simulink model "templateVFreplay"  (R2019b)
settings: Solver=ode23tb  StartTime=0  StopTime=dataSim(l).Time(end)  FixedStep=Ts
model workspace (MAT data in the model file):
  AC8B_test_sdosession : sldodialogs.data.SessionData (value not decoded)
  tp34291882_bceb_4da8_b486_81ba615ab517 = [0 0.0333333 0.0666667 0.1 0.1333334 0.1666667 0.2 0.2333333 0.2666666 0.2999999 0.3333332 0.3666665 ... (13500 elements, 2700x5)]
  tp5fd81924_c6b2_4820_a4c1_c746ac51258e : object (value not decoded)
  tp61e2f470_2812_498a_af75_e87b8b944307 = [0 0.0333333 0.0666667 0.1 0.1333334 0.1666667 0.2 0.2333333 0.2666666 0.2999999 0.3333332 0.3666665 ... (13500 elements, 2700x5)]
  tpfa3056f0_c430_45b3_969f_b76cef1498ad : object (value not decoded)
undefined symbols (not defined in the file): dataSim, dyn, Fnom, g, gcbh, genTpd0, genTppd0, genTppq0, genTpq0, genXd, genXl, genXpd, genXppd, genXppq, genXpq, genXq, govDisable, ifd, init, j, l, MBase, p, sps_rtmsupport, sys, Tb1, Tc1, Vnom, vt
libraries: powerlib x28, modelLibrary x22, simulink x15, powerlib_meascontrol x5, spsST2AModel x4, GenLib x2, ideal_source x1
(part 3 of 4)

== system templateVFreplay/VF Replay/GOV/IEEEG3 ==
  Pref : Inport
  meas : Inport  Port=2
  Bus Selector10 : BusSelector  OutputSignals="Mechanical.Rotor speed  wm  (pu),Mechanical.Electrical power  Pe (pu)"
  Hydro Turbine/Governor (Continuous) : Subsystem  mask(IEEEG3 Hydro Turbine/Governor Model){Tg=p.tg, Tp=p.tp, Uo=p.uo, Uc=p.uc, Pmax=p.pmax, Pmin=p.pmin, Rperm=p.rperm, Rtemp=p.rtemp, Tr=p.tr, Tw=p.tw, Kturb=p.kturb, Aturb=p.aturb, Bturb=p.bturb, db1=p.db1, eps=p.eps, db2=p.db2, Gv=[p.gv1 p.gv2 p.gv3 p.gv4 p.gv5 p.gv6], Pgv=[p.pgv1 p.pgv2 p.pgv3 p.pgv4 p.pgv5 p.pgv6]}
      mask prompts: Tg "Tg, Gate servo time constant [s]"; Tp "Tp, Pilot servo time constant [s]"; Uo "Uo, Maximum gate opening rate [pu/sec]"; Uc "Uc, Maximum gate closing rate [pu/s]"; Pmax "Pmax, Max gate opening [pu of mw]"; Pmin "Pmin, Minimum gate opening [pu of mx]"; Rperm "Rperm, Permanent droop [pu]"; Rtemp "Rtemp, Temporary droop [pu]"; Tr "Tr, Dashpot time constant [s]"; Tw "Tw, Water inertia time constant [s]"; Kturb "Kturb, Turbine gain [pu]"; Aturb "Aturb, Turbine numerator"; Bturb "Bturb, Turbine denominator"; db1 "db1, Intentional deadband width, Hz"; eps "eps, Intentional deadband hysteresis, Hz"; db2 "db2, Unintentional deadband [MW]"; Gv "Gv, Nonlinear Gain Points [Gv1 Gv2 Gv3 Gv4 Gv5 Gv6], [pu]"; Pgv "Pgv, Nonlinear Gain Points [Pgv1 Pgv2 Pgv3 Pgv4 Pgv5 Pgv6], [pu]"
      mask DialogControl Container9 Prompt: Gate
      mask DialogControl Container11 Prompt: Droop
      mask DialogControl Container12 Prompt: Turbine
      mask DialogControl Container13 Prompt: Nonlinear Effects
      mask Display:
      | port_label('input',1,'Pref');
      | port_label('input',2,'Speed');
      | port_label('output',1,'Pmech');
      | 
      | color('blue');disp('IEEEG3')
  Terminator : Terminator
  Pm : Outport  VectorParamsAs1DForOutWhenUnconnected=off
  wires:
  meas/1 -> Bus Selector10/1
  Pref/1 -> Hydro Turbine/Governor (Continuous)/1(Pref)
  Bus Selector10/2 -> Terminator/1  "<Electrical power  Pe (pu)>"
  Hydro Turbine/Governor (Continuous)/1(Pmech) -> Pm/1
  Bus Selector10/1 -> Hydro Turbine/Governor (Continuous)/2(Speed)  "<Rotor speed  wm  (pu)>"

== system templateVFreplay/VF Replay/PSS/PSS1A ==
  meas : Inport
  Bus Selector9 : BusSelector  OutputSignals="Mechanical.Rotor speed deviation  dw (pu),Mechanical.Electrical power  Pe (pu)"
  Power System Stabilize 1A (Continuous) : Subsystem  mask(PSS1A - Single Input Power System Stabilizer){A1=p.a1, A2=p.a2, T1=p.t1, T2=p.t2, T3=p.t3, T4=p.t4, T5=p.t5, T6=p.t6, Ks=p.ks, Vrmax=p.vrmax, Vrmin=p.vrmin}
      mask prompts: A1 "A1, Notch filter parameter"; A2 "A2, Notch filter parameter"; T1 "T1, Lead/lag time constant [s]"; T2 "T2, Lead/lag time constant [s]"; T3 "T3, Lead/lag time constant [s]"; T4 "T4, Lead/lag time constant [s]"; T5 "T5, Washout time constant [s]"; T6 "T6, Transducer time constant [s]"; Ks "Ks, Stabilizer gain"; Vrmax "Vrmax, Maximum stabilizer output [pu]"; Vrmin "Vrmin, Minimize stabilizer output [pu]"
      mask DialogControl Container9 Prompt: Filter Time Constants
      mask DialogControl Container11 Prompt: Stabilizer
      mask Display:
      | port_label('input',1,'Input');
      | port_label('output',1,'Vstab');
      | 
      | color('blue');disp('PSS1A')
  Terminator : Terminator
  Vstab : Outport  VectorParamsAs1DForOutWhenUnconnected=off
  wires:
  Bus Selector9/2 -> Terminator/1  "<Electrical power  Pe (pu)>"
  Bus Selector9/1 -> Power System Stabilize 1A (Continuous)/1(Input)  "<Rotor speed deviation  dw (pu)>"
  Power System Stabilize 1A (Continuous)/1(Vstab) -> Vstab/1
  meas/1 -> Bus Selector9/1

== system templateVFreplay/VF Replay/PSS/PSS2A ==
  meas : Inport
  Bus Selector9 : BusSelector  OutputSignals="Mechanical.Rotor speed  wm  (pu),Mechanical.Electrical power  Pe (pu)"
  "Power System Stabilizer 2A (Continuous) " : Subsystem  mask(PSS2A - Duel Input Power System Stabilizer){TwSig1=[p.tw1 p.tw2], TwSig2=[p.tw3 p.tw4], T12=[p.t1 p.t2], T34=[p.t3 p.t4], T6=p.t6, T7=p.t7, T89=[p.t8 p.t9], Order=[p.n p.m], Tab=[p.a p.ta p.tb], Ks1=p.ks1, KsVec=[p.ks2 p.ks3 p.ks4], Vstmax=p.vstmax, Vstmin=p.vstmin}
      mask prompts: TwSig1 "[Tw1 Tw2], Washout Parameters, Signal #1"; TwSig2 "[Tw3 Tw4], Washout Parameters, Signal #2 [s]"; T12 "[T1 T2], Lead/lag time constant [s]"; T34 "[T3 T4], Lead/lag time constant [s]"; T6 "T6, Time Constant, Signal #1 [s]"; T7 "T7, Time Constant, Signal #2 [s]"; T89 "[T8 T9], Lead/Lag Ramp Tracking"; Order "[n m], Order of Tracking Filter"; Tab "[a Ta Tb], Gain/Lead/Lag Time Constants"; Ks1 "Ks1, Stabilizer Gain"; KsVec "[Ks2 Ks3 Ks4], Signal #2 Gains"; Vstmax "Vstmax, Maximum stabilizer output [pu]"; Vstmin "Vstmin, Minimize stabilizer output [pu]"
      mask init:
      | Tw1 = TwSig1(1);    Tw2 = TwSig1(2);
      | Tw3 = TwSig2(1);    Tw4 = TwSig2(2);
      | T1 = T12(1);        T2 = T12(2);
      | T3 = T34(1);        T4 = T34(2);
      | T8 = T89(1);        T9 = T89(2);
      | N = Order(1);       M = Order(2);
      | a = Tab(1);         Ta = Tab(2);        Tb = Tab(3);
      | Ks2 = KsVec(1);     Ks3 = KsVec(2);     Ks4 = KsVec(3);
      mask DialogControl Container9 Prompt: Filter Time Constants
      mask DialogControl Container11 Prompt: Stabilizer
      mask Display:
      | port_label('input',1,'Input 1');
      | port_label('input',2,'Input 2');
      | port_label('output',1,'Vstab');
      | 
      | color('blue');disp('PSS2A')
  Vstab : Outport  VectorParamsAs1DForOutWhenUnconnected=off
  wires:
  meas/1 -> Bus Selector9/1
  "Power System Stabilizer 2A (Continuous) "/1(Vstab) -> Vstab/1
  Bus Selector9/1 -> "Power System Stabilizer 2A (Continuous) "/1(Input_1)  "<Rotor speed  wm  (pu)>"
  Bus Selector9/2 -> "Power System Stabilizer 2A (Continuous) "/2(Input_2)  "<Electrical power  Pe (pu)>"

== system templateVFreplay/VF Replay/PSS/PSS2B ==
  meas : Inport
  Bus Selector3 : BusSelector  OutputSignals="Mechanical.Rotor speed deviation  dw (pu),Mechanical.Electrical power  Pe (pu)"
  "Power System Stabilizer 2B (Continuous) " : Subsystem  mask(PSS2A - Duel Input Power System Stabilizer){TwSig1=[p.tw1 p.tw2], TwSig2=[p.tw3 p.tw4], T12=[p.t1 p.t2], T34=[p.t3 p.t4], T6=p.t6, T7=p.t7, T89=[p.t8 p.t9], Order=[p.n p.m], Tab=[p.a p.ta p.tb], Ks1=p.ks1, KsVec=[p.ks2 p.ks3 p.ks4], Vstmax=p.vstmax, Vstmin=p.vstmin}
      mask prompts: TwSig1 "[Tw1 Tw2], Washout Parameters, Signal #1"; TwSig2 "[Tw3 Tw4], Washout Parameters, Signal #2 [s]"; T12 "[T1 T2], Lead/lag time constant [s]"; T34 "[T3 T4], Lead/lag time constant [s]"; T6 "T6, Time Constant, Signal #1 [s]"; T7 "T7, Time Constant, Signal #2 [s]"; T89 "[T8 T9], Lead/Lag Ramp Tracking"; Order "[n m], Order of Tracking Filter"; Tab "[a Ta Tb], Gain/Lead/Lag Time Constants"; Ks1 "Ks1, Stabilizer Gain"; KsVec "[Ks2 Ks3 Ks4], Signal #2 Gains"; Vstmax "Vstmax, Maximum stabilizer output [pu]"; Vstmin "Vstmin, Minimize stabilizer output [pu]"
      mask init: same as templateVFreplay/VF Replay/PSS/PSS2A/Power System Stabilizer 2A (Continuous) 
      mask DialogControl Container9 Prompt: Filter Time Constants
      mask DialogControl Container11 Prompt: Stabilizer
      mask Display:
      | port_label('input',1,'Input 1');
      | port_label('input',2,'Input 2');
      | port_label('output',1,'Vstab');
      | 
      | color('blue');disp('PSS2B')
  Vstab : Outport  VectorParamsAs1DForOutWhenUnconnected=off
  wires:
  Bus Selector3/2 -> "Power System Stabilizer 2B (Continuous) "/2(Input_2)  "<Electrical power  Pe (pu)>"
  Bus Selector3/1 -> "Power System Stabilizer 2B (Continuous) "/1(Input_1)  "<Rotor speed deviation  dw (pu)>"
  meas/1 -> Bus Selector3/1
  "Power System Stabilizer 2B (Continuous) "/1(Vstab) -> Vstab/1

== system templateVFreplay/VF Replay/Subsystem/PQ VF ==
  u : Inport
  Constant1 : Constant  Value=[dataSim(l).Pact(1) dataSim(l).Qact(1)]
  GainPQgo : Gain  Gain=[1/dataSim(l).maxP 1/dataSim(l).maxQ]
  Sum1 : Sum  Inputs=|+-
  y : Outport  SampleTime=1/30  VectorParamsAs1DForOutWhenUnconnected=off
  tag scope: PQgoVF=global
  wires:
  u/1 -> Sum1/1
  GainPQgo/1 -> [PQgoVF], y/1
  Sum1/1 -> GainPQgo/1
  Constant1/1 -> Sum1/2

== system templateVFreplay/VF Replay/Subsystem/PQ VF comp ==
  u : Inport
  From Workspace3 : FromWorkspace  VariableName=[dataSim(l).Time dataSim(l).Pact dataSim(l).Qact]  SampleTime=0
  Mux2 : Mux  Inputs=2
  To File4 : ToFile  Filename=PQsVF.mat  MatrixName=PQVF  SaveFormat=Timeseries  SampleTime=1/30
  "y " : Outport  VectorParamsAs1DForOutWhenUnconnected=off
  wires:
  u/1 -> Mux2/2
  Mux2/1 -> "y "/1, To File4/1
  From Workspace3/1 -> Mux2/1

== system templateVFreplay/VF Replay/Subsystem/V VF comp ==
  u : Inport
  From Workspace5 : FromWorkspace  VariableName=[dataSim(l).Time dataSim(l).Vact]  SampleTime=0
  Mux6 : Mux  Inputs=2
  To File5 : ToFile  Filename=vsVF.mat  MatrixName=vVF  SaveFormat=Timeseries
  y : Outport  VectorParamsAs1DForOutWhenUnconnected=off
  wires:
  u/1 -> Mux6/2
  From Workspace5/1 -> Mux6/1
  Mux6/1 -> y/1, To File5/1

== system templateVFreplay/VF Replay/Subsystem/VF VF ==
  u : Inport
  Constant : Constant  Value=[dataSim(l).Vact(1)/Vnom dataSim(l).Fact(1)/Fnom]
  Gain5 : Gain  Gain=1/500
  Gainvwo : Gain  Gain=[1/dataSim(l).maxF 1/dataSim(l).maxV]
  Selector1 : Selector  InputPortWidth=2  IndexOptions=Index vector (dialog)  Indices=[2 1]  OutputSizes=1
  Sum : Sum  Inputs=|+-
  muxvw : Mux  Inputs=2
  y : Outport  VectorParamsAs1DForOutWhenUnconnected=off
  wires:
  u/1 -> Gain5/1
  Gainvwo/1 -> y/1
  Gain5/1 -> muxvw/1
  Sum/1 -> Selector1/1
  muxvw/1 -> Sum/1
  Constant/1 -> Sum/2
  Selector1/1 -> Gainvwo/1
  [woVF] -> muxvw/2

== system templateVFreplay/VF Replay/Subsystem/freq ==
  From Workspace4 : FromWorkspace  VariableName=[dataSim(l).Time dataSim(l).Fact/Fnom]  SampleTime=0
  Mux5 : Mux  Inputs=2
  To File3 : ToFile  Filename=wsVF.mat  MatrixName=wVF  SaveFormat=Timeseries
  y : Outport  VectorParamsAs1DForOutWhenUnconnected=off
  wires:
  Mux5/1 -> y/1, To File3/1
  From Workspace4/1 -> Mux5/1
  [fGridVF] -> Mux5/2

== system templateVFreplay/VF Replay/meas VF/Euclidian Norm5 ==
  u1 : Inport
  u2 : Inport  Port=2
  Math Function : Math  Operator=square  SaturateOnIntegerOverflow=on
  Mux : Mux  Inputs=2
  Sqrt : Sqrt  SaturateOnIntegerOverflow=on
  Sum of Elements : Sum  Inputs=+
  y : Outport  VectorParamsAs1DForOutWhenUnconnected=off
  wires:
  Sqrt/1 -> y/1
  Mux/1 -> Math Function/1
  u2/1 -> Mux/2
  u1/1 -> Mux/1
  Math Function/1 -> Sum of Elements/1
  Sum of Elements/1 -> Sqrt/1

== system templateVFreplay/VF Replay/meas VF/wo VF ==
  u : Inport
  Gainwo : Gain
  y : Outport  VectorParamsAs1DForOutWhenUnconnected=off
  tag scope: woVF=global
  wires:
  u/1 -> Gainwo/1
  Gainwo/1 -> y/1, [woVF]

== system templateVFreplay/VF Replay/AVR/REXS/Euclidian Norm3 ==
  u1 : Inport
  u2 : Inport  Port=2
  Math Function : Math  Operator=square  SaturateOnIntegerOverflow=on
  Mux : Mux  Inputs=2
  Sqrt : Sqrt  SaturateOnIntegerOverflow=on
  Sum of Elements : Sum  Inputs=+
  y : Outport  VectorParamsAs1DForOutWhenUnconnected=off
  wires:
  Sqrt/1 -> y/1
  Mux/1 -> Math Function/1
  u2/1 -> Mux/2
  u1/1 -> Mux/1
  Math Function/1 -> Sum of Elements/1
  Sum of Elements/1 -> Sqrt/1

== system templateVFreplay/VF Replay/AVR/REXS/Euclidian Norm4 ==
  u1 : Inport
  u2 : Inport  Port=2
  Math Function : Math  Operator=square  SaturateOnIntegerOverflow=on
  Mux : Mux  Inputs=2
  Sqrt : Sqrt  SaturateOnIntegerOverflow=on
  Sum of Elements : Sum  Inputs=+
  y : Outport  VectorParamsAs1DForOutWhenUnconnected=off
  wires:
  Sum of Elements/1 -> Sqrt/1
  Math Function/1 -> Sum of Elements/1
  u1/1 -> Mux/1
  u2/1 -> Mux/2
  Mux/1 -> Math Function/1
  Sqrt/1 -> y/1

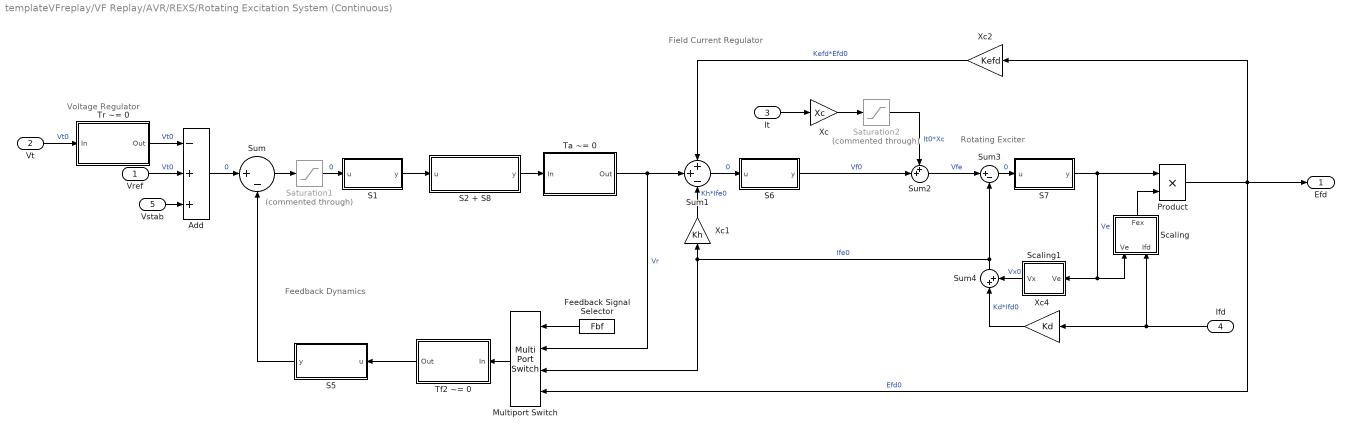
== system templateVFreplay/VF Replay/AVR/REXS/Rotating Excitation System (Continuous)  ==
  note: Voltage Regulator
  note: Rotating Exciter
  note: Feedback Dynamics
  note: Field Current Regulator
  Vref : Inport
  Vt : Inport  Port=2
  It : Inport  Port=3
  Ifd : Inport  Port=4
  Vstab : Inport  Port=5
  Add : Sum  Inputs=-++
  Feedback Signal Selector : Constant  Value=Fbf
  Multiport Switch : MultiPortSwitch  DataPortOrder=Zero-based contiguous  zeroidx=on
  Product : Product
  S1 : Subsystem
      mask Display: disp('K_{vp} + K_{vi}/s','texmode','on');
  S2 + S8 : Subsystem
      mask Display: disp('(1 + s T_{c1})(1 + s T_{c2})/(1 + s T_{b1})(1 + s T_{b2})','texmode','on');
  S5 : Subsystem
      mask Display: disp('s K_f / (1 + s T_f)','texmode','on');
  S6 : Subsystem
      mask Display: disp('K_{ip} + K_{ii}/s','texmode','on');
  S7 : Subsystem
      mask Display: disp('1/(s T_e)','texmode','on');
  Saturation1 : Saturate  Commented=through  UpperLimit=Vimax  LowerLimit=-Vimax
      settings: AttributesFormatString=|
      | %<UpperLimit>
      | %<LowerLimit>
  Saturation2 : Saturate  Commented=through  UpperLimit=Vcmax  LowerLimit=-Inf
      settings: AttributesFormatString=|
      | %<UpperLimit>
      | %<LowerLimit>
  Scaling : Subsystem
      mask Display: disp('F(I_{fd},V_e)','texmode','on');
  Scaling1 : Subsystem
      mask Display: disp('K_e + S_e','texmode','on');
  Sum : Sum  Inputs=|+-
  Sum1 : Sum  Inputs=++-
  Sum2 : Sum  Inputs=++|
  Sum3 : Sum  Inputs=|+-
  Sum4 : Sum  Inputs=|++
  Ta ~= 0 : Subsystem  VariantControl=TaNotZero
  Tf2 ~= 0 : Subsystem  VariantControl=Tf2NotZero
  Tr ~= 0 : Subsystem  VariantControl=TrNotZero
  Xc : Gain  Gain=Xc
  Xc1 : Gain  Gain=Kh
  Xc2 : Gain  Gain=Kefd
  Xc4 : Gain  Gain=Kd
  Efd : Outport  VectorParamsAs1DForOutWhenUnconnected=off
  wires:
  It/1 -> Xc/1
  Ifd/1 -> Scaling/2(Ifd), Xc4/1
  S5/1(y) -> Sum/2
  Tf2 ~= 0/1(Out) -> S5/1(u)
  Multiport Switch/1 -> Tf2 ~= 0/1(In)
  Feedback Signal Selector/1 -> Multiport Switch/1
  Scaling/1(Fex) -> Product/2
  Xc4/1 -> Sum4/1  "Kd*Ifd0"
  S7/1(y) -> Scaling/1(Ve), Scaling1/1(Ve), Product/1  "Ve"
  Scaling1/1(Vx) -> Sum4/2  "Vx0"
  Product/1 -> Multiport Switch/4, Efd/1, Xc2/1  "Efd0"
  Xc2/1 -> Sum1/1  "Kefd*Efd0"
  Xc1/1 -> Sum1/3  "Kh*Ife0"
  Sum4/1 -> Sum3/2, Multiport Switch/3, Xc1/1  "Ife0"
  Sum3/1 -> S7/1(u)  "0"
  Sum2/1 -> Sum3/1  "Vfe"
  Saturation2/1 -> Sum2/1  "It0*Xc"
  Xc/1 -> Saturation2/1
  S6/1(y) -> Sum2/2  "Vf0"
  Sum1/1 -> S6/1(u)  "0"
  Ta ~= 0/1(Out) -> Sum1/2, Multiport Switch/2  "Vr"
  S2 + S8/1(y) -> Ta ~= 0/1(In)
  S1/1(y) -> S2 + S8/1(u)
  Saturation1/1 -> S1/1(u)  "0"
  Sum/1 -> Saturation1/1
  Add/1 -> Sum/1  "0"
  Vstab/1 -> Add/3
  Vref/1 -> Add/2  "Vt0"
  Tr ~= 0/1(Out) -> Add/1  "Vt0"
  Vt/1 -> Tr ~= 0/1(In)  "Vt0"

== system templateVFreplay/VF Replay/AVR/ST1A/Euclidian Norm1 ==
  u : Inport
  Math Function : Math  Operator=square  SaturateOnIntegerOverflow=on
  Sqrt : Sqrt  SaturateOnIntegerOverflow=on
  Sum of Elements : Sum  Inputs=+
  y : Outport  VectorParamsAs1DForOutWhenUnconnected=off
  wires:
  Sum of Elements/1 -> Sqrt/1
  Math Function/1 -> Sum of Elements/1
  Sqrt/1 -> y/1  "t"
  u/1 -> Math Function/1

== system templateVFreplay/VF Replay/AVR/ST1A/ST1A Excitation System ==
  Vref : Inport
  Vt : Inport  Port=2
  Ifd : Inport  Port=3
  Vstab : Inport  Port=4
  Model : Subsystem  mask(Excitation System){}
  Efd : Outport  VectorParamsAs1DForOutWhenUnconnected=off
  wires:
  Vstab/1 -> Model/4(Vstab)
  Ifd/1 -> Model/3(Ifd)
  Vref/1 -> Model/1(Vref)
  Vt/1 -> Model/2(Vt)
  Model/1(Efd) -> Efd/1

== system templateVFreplay/VF Replay/AVR/ST4B/Euclidian Norm ==
  u : Inport
  Math Function : Math  Operator=square  SaturateOnIntegerOverflow=on
  Sqrt : Sqrt  SaturateOnIntegerOverflow=on
  Sum of Elements : Sum  Inputs=+
  y : Outport  VectorParamsAs1DForOutWhenUnconnected=off
  wires:
  u/1 -> Math Function/1
  Sqrt/1 -> y/1  "t"
  Math Function/1 -> Sum of Elements/1
  Sum of Elements/1 -> Sqrt/1

== system templateVFreplay/VF Replay/AVR/ST4B/Euclidian Norm1 ==
  u : Inport
  Math Function : Math  Operator=square  SaturateOnIntegerOverflow=on
  Sqrt : Sqrt  SaturateOnIntegerOverflow=on
  Sum of Elements : Sum  Inputs=+
  y : Outport  VectorParamsAs1DForOutWhenUnconnected=off
  wires:
  u/1 -> Math Function/1
  Sqrt/1 -> y/1  "t"
  Math Function/1 -> Sum of Elements/1
  Sum of Elements/1 -> Sqrt/1

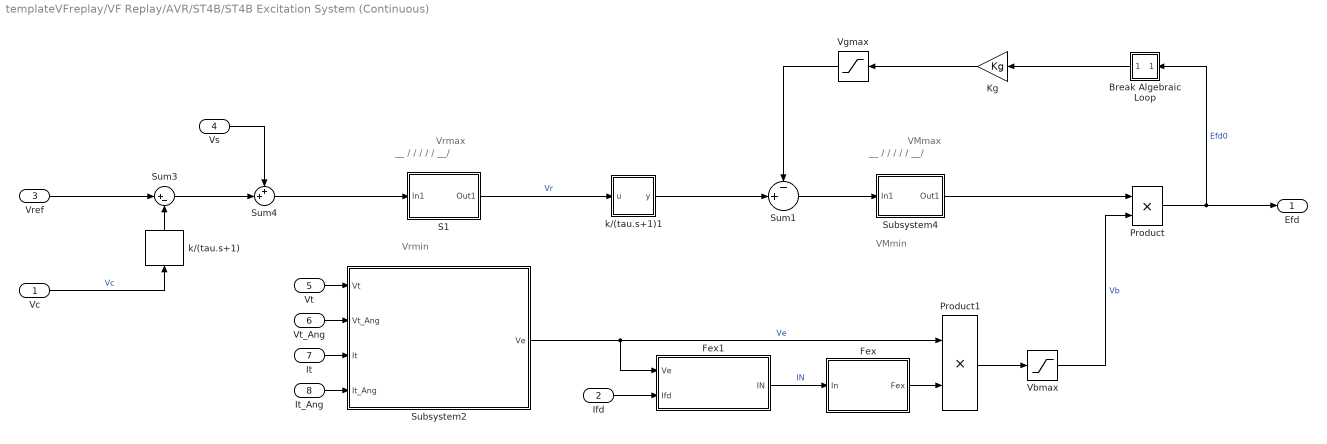
== system templateVFreplay/VF Replay/AVR/ST4B/ST4B Excitation System (Continuous) ==
  note: __
      |               /
      |             /
      |           /
      |         /
      |       /
      | __/
  note: Vrmax
  note: Vrmin
  note: __
      |               /
      |             /
      |           /
      |         /
      |       /
      | __/
  note: VMmax
  note: VMmin
  Vc : Inport
  Ifd : Inport  Port=2
  Vref : Inport  Port=3
  Vs : Inport  Port=4
  Vt : Inport  Port=5
  Vt_Ang : Inport  Port=6
  It : Inport  Port=7
  It_Ang : Inport  Port=8
  "Break Algebraic Loop " : Subsystem
      mask Display: disp('1 / (1 + s T_{pelec})','texmode','on');
  Fex : Subsystem
      mask Display: disp('Fex = f(IN)');
  Fex1 : Subsystem  mask{Kc=Kc}
      mask prompts: Kc "Exciter regulation factor, Kc(pu):"
      mask Display: disp('In = Kc*Ifd/Ve')
  Kg : Gain  Gain=Kg
  Product : Product  SaturateOnIntegerOverflow=on  RndMeth=Zero  InputSameDT=on  OutDataTypeStr=Inherit: Same as first input
  Product1 : Product  SaturateOnIntegerOverflow=on  RndMeth=Zero  InputSameDT=on  OutDataTypeStr=Inherit: Same as first input
  S1 : Subsystem
      mask Display: disp('K_{pr} + K_{ir}/s','texmode','on');
  Subsystem2 : Subsystem
      mask Display: disp('Ve = |Kp*Vt+j(Ki+Kp*XL)*It|')
  Subsystem4 : Subsystem
      mask Display: disp('K_{pm} + K_{im}/s','texmode','on');
  Sum1 : Sum  Inputs=-+|
  Sum3 : Sum  Inputs=|+-
  Sum4 : Sum  Inputs=++|
  Vbmax : Saturate  UpperLimit=Vbmax  LowerLimit=-inf
  Vgmax : Saturate  UpperLimit=Vgmax  LowerLimit=-inf
  k/(tau.s+1) : modelLibrary/k//(tau.s+1)  k=1  tau=Tr  vmax=Inf  vmin=-Inf
  k/(tau.s+1)1 : Subsystem  mask{k=1, tau=Ta, vmax=Inf, vmin=-Inf}
  Efd : Outport  VectorParamsAs1DForOutWhenUnconnected=off
  wires:
  Vref/1 -> Sum3/1
  k/(tau.s+1)/1 -> Sum3/2
  Vs/1 -> Sum4/1
  Sum3/1 -> Sum4/2
  Vc/1 -> k/(tau.s+1)/1  "Vc"
  Product/1 -> Efd/1, "Break Algebraic Loop "/1(In)  "Efd0"
  It/1 -> Subsystem2/3(It)
  Vbmax/1 -> Product/2  "Vb"
  Subsystem2/1(Ve) -> Product1/1, Fex1/1(Ve)  "Ve"
  Sum4/1 -> S1/1(In1)
  Sum1/1 -> Subsystem4/1(In1)
  Kg/1 -> Vgmax/1
  Product1/1 -> Vbmax/1
  Vt/1 -> Subsystem2/1(Vt)
  Vt_Ang/1 -> Subsystem2/2(Vt_Ang)
  Fex1/1(IN) -> Fex/1(In)  "IN"
  Fex/1(Fex) -> Product1/2
  It_Ang/1 -> Subsystem2/4(It_Ang)
  Ifd/1 -> Fex1/2(Ifd)
  Vgmax/1 -> Sum1/1
  "Break Algebraic Loop "/1(Out) -> Kg/1
  k/(tau.s+1)1/1(y) -> Sum1/2
  S1/1(Out1) -> k/(tau.s+1)1/1(u)  "Vr"
  Subsystem4/1(Out1) -> Product/1

== system templateVFreplay/VF Replay/AVR/ST4B/Subsystem1 ==
  u : Inport
  Demux : Demux  Outputs=2
  Divide : Product  Inputs=*/
  Trigonometric Function : Trigonometry  Operator=atan
  y : Outport  VectorParamsAs1DForOutWhenUnconnected=off
  wires:
  Demux/1 -> Divide/1
  u/1 -> Demux/1
  Demux/2 -> Divide/2
  Trigonometric Function/1 -> y/1
  Divide/1 -> Trigonometric Function/1

== system templateVFreplay/VF Replay/AVR/ST4B/Subsystem2 ==
  u : Inport
  Demux : Demux  Outputs=2
  Divide : Product  Inputs=*/
  Trigonometric Function : Trigonometry  Operator=atan
  y : Outport  VectorParamsAs1DForOutWhenUnconnected=off
  wires:
  Demux/1 -> Divide/1
  u/1 -> Demux/1
  Demux/2 -> Divide/2
  Trigonometric Function/1 -> y/1
  Divide/1 -> Trigonometric Function/1

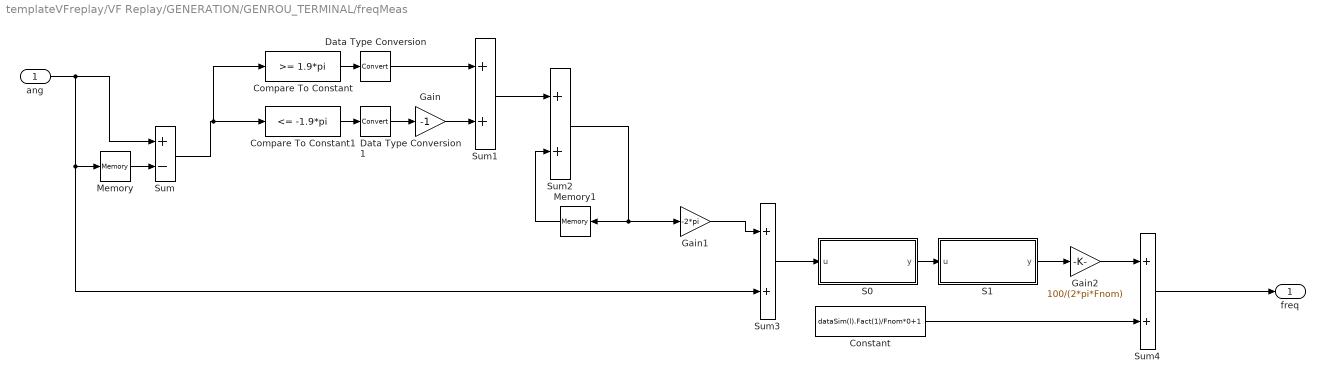
== system templateVFreplay/VF Replay/GENERATION/GENROU_TERMINAL/freqMeas ==
  ang : Inport
  Compare To Constant : simulink/Logic and Bit Operations/Compare To Constant  relop=>=  const=1.9*pi  OutDataTypeStr=boolean
  Compare To Constant1 : simulink/Logic and Bit Operations/Compare To Constant  relop=<=  const=-1.9*pi  OutDataTypeStr=boolean
  Constant : Constant  Value=dataSim(l).Fact(1)/Fnom*0+1
  Data Type Conversion : DataTypeConversion
  Data Type Conversion1 : DataTypeConversion
  Gain : Gain  Gain=-1
  Gain1 : Gain  Gain=-2*pi
  Gain2 : Gain  Gain=100/(2*pi*Fnom)
  Memory : Memory  InheritSampleTime=on
  Memory1 : Memory  InheritSampleTime=on
  S0 : Subsystem
      mask Display: disp('s T_{w1} / (1 + s T_{w1})','texmode','on');
  S1 : Subsystem
      mask Display: disp('1/ (1 + s T)','texmode','on');
  Sum : Sum  Inputs=+-
  Sum{1..4} (4 alike) : Sum
  freq : Outport  VectorParamsAs1DForOutWhenUnconnected=off
  wires:
  Sum4/1 -> freq/1
  Gain2/1 -> Sum4/1
  Constant/1 -> Sum4/2
  Sum3/1 -> S0/1(u)
  Gain1/1 -> Sum3/1
  Data Type Conversion1/1 -> Gain/1
  Data Type Conversion/1 -> Sum1/1
  Memory/1 -> Sum/2
  Memory1/1 -> Sum2/2
  Gain/1 -> Sum1/2
  S0/1(y) -> S1/1(u)
  Compare To Constant/1 -> Data Type Conversion/1
  Compare To Constant1/1 -> Data Type Conversion1/1
  Sum2/1 -> Memory1/1, Gain1/1
  Sum/1 -> Compare To Constant1/1, Compare To Constant/1
  Sum1/1 -> Sum2/1
  ang/1 -> Sum3/2, Memory/1, Sum/1
  S1/1(y) -> Gain2/1

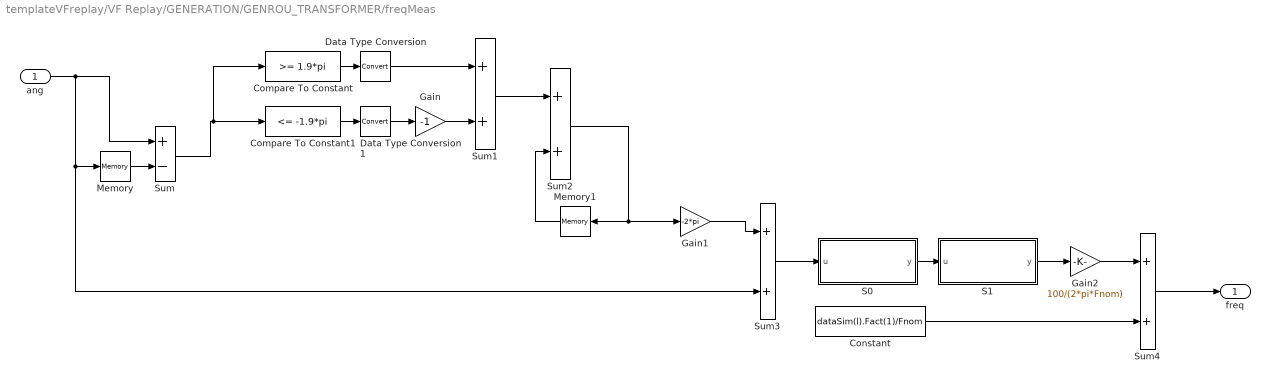
== system templateVFreplay/VF Replay/GENERATION/GENROU_TRANSFORMER/freqMeas ==
  ang : Inport
  Compare To Constant : simulink/Logic and Bit Operations/Compare To Constant  relop=>=  const=1.9*pi  OutDataTypeStr=boolean
  Compare To Constant1 : simulink/Logic and Bit Operations/Compare To Constant  relop=<=  const=-1.9*pi  OutDataTypeStr=boolean
  Constant : Constant  Value=dataSim(l).Fact(1)/Fnom
  Data Type Conversion : DataTypeConversion
  Data Type Conversion1 : DataTypeConversion
  Gain : Gain  Gain=-1
  Gain1 : Gain  Gain=-2*pi
  Gain2 : Gain  Gain=100/(2*pi*Fnom)
  Memory : Memory  InheritSampleTime=on
  Memory1 : Memory  InheritSampleTime=on
  S0 : Subsystem
      mask Display: disp('s T_{w1} / (1 + s T_{w1})','texmode','on');
  S1 : Subsystem
      mask Display: disp('1/ (1 + s T)','texmode','on');
  Sum : Sum  Inputs=+-
  Sum{1..4} (4 alike) : Sum
  freq : Outport  VectorParamsAs1DForOutWhenUnconnected=off
  wires:
  S1/1(y) -> Gain2/1
  ang/1 -> Sum/1, Memory/1, Sum3/2
  Sum1/1 -> Sum2/1
  Sum/1 -> Compare To Constant/1, Compare To Constant1/1
  Sum2/1 -> Gain1/1, Memory1/1
  Compare To Constant1/1 -> Data Type Conversion1/1
  Compare To Constant/1 -> Data Type Conversion/1
  S0/1(y) -> S1/1(u)
  Gain/1 -> Sum1/2
  Memory1/1 -> Sum2/2
  Memory/1 -> Sum/2
  Data Type Conversion/1 -> Sum1/1
  Data Type Conversion1/1 -> Gain/1
  Gain1/1 -> Sum3/1
  Sum3/1 -> S0/1(u)
  Constant/1 -> Sum4/2
  Gain2/1 -> Sum4/1
  Sum4/1 -> freq/1

== system templateVFreplay/VF Replay/GENERATION/GENSAL_TRANSFORMER/freqMeas ==
  ang : Inport
  Compare To Constant : simulink/Logic and Bit Operations/Compare To Constant  relop=>=  const=1.9*pi  OutDataTypeStr=boolean
  Compare To Constant1 : simulink/Logic and Bit Operations/Compare To Constant  relop=<=  const=-1.9*pi  OutDataTypeStr=boolean
  Constant : Constant  Value=dataSim(l).Fact(1)/Fnom
  Data Type Conversion : DataTypeConversion
  Data Type Conversion1 : DataTypeConversion
  Gain : Gain  Gain=-1
  Gain1 : Gain  Gain=-2*pi
  Gain2 : Gain  Gain=100/(2*pi*Fnom)
  Memory : Memory  InheritSampleTime=on
  Memory1 : Memory  InheritSampleTime=on
  S0 : Subsystem
      mask Display: disp('s T_{w1} / (1 + s T_{w1})','texmode','on');
  S1 : Subsystem
      mask Display: disp('1/ (1 + s T)','texmode','on');
  Sum : Sum  Inputs=+-
  Sum{1..4} (4 alike) : Sum
  freq : Outport  VectorParamsAs1DForOutWhenUnconnected=off
  wires:
  Sum4/1 -> freq/1
  Gain2/1 -> Sum4/1
  Constant/1 -> Sum4/2
  Sum3/1 -> S0/1(u)
  Gain1/1 -> Sum3/1
  Data Type Conversion1/1 -> Gain/1
  Data Type Conversion/1 -> Sum1/1
  Memory/1 -> Sum/2
  Memory1/1 -> Sum2/2
  Gain/1 -> Sum1/2
  S0/1(y) -> S1/1(u)
  Compare To Constant/1 -> Data Type Conversion/1
  Compare To Constant1/1 -> Data Type Conversion1/1
  Sum2/1 -> Memory1/1, Gain1/1
  Sum/1 -> Compare To Constant1/1, Compare To Constant/1
  Sum1/1 -> Sum2/1
  ang/1 -> Sum3/2, Memory/1, Sum/1
  S1/1(y) -> Gain2/1

== system templateVFreplay/VF Replay/GENERATION/GENTPJ_TERMINAL/freqMeas ==
  ang : Inport
  Compare To Constant : simulink/Logic and Bit Operations/Compare To Constant  relop=>=  const=1.9*pi  OutDataTypeStr=boolean
  Compare To Constant1 : simulink/Logic and Bit Operations/Compare To Constant  relop=<=  const=-1.9*pi  OutDataTypeStr=boolean
  Constant : Constant  Value=dataSim(l).Fact(1)/Fnom
  Data Type Conversion : DataTypeConversion
  Data Type Conversion1 : DataTypeConversion
  Gain : Gain  Gain=-1
  Gain1 : Gain  Gain=-2*pi
  Gain2 : Gain  Gain=100/(2*pi*Fnom)
  Memory : Memory  InheritSampleTime=on
  Memory1 : Memory  InheritSampleTime=on
  S0 : Subsystem
      mask Display: disp('s T_{w1} / (1 + s T_{w1})','texmode','on');
  S1 : Subsystem
      mask Display: disp('1/ (1 + s T)','texmode','on');
  Sum : Sum  Inputs=+-
  Sum{1..4} (4 alike) : Sum
  freq : Outport  VectorParamsAs1DForOutWhenUnconnected=off
  wires:
  Sum4/1 -> freq/1
  Gain2/1 -> Sum4/1
  Constant/1 -> Sum4/2
  Sum3/1 -> S0/1(u)
  Gain1/1 -> Sum3/1
  Data Type Conversion1/1 -> Gain/1
  Data Type Conversion/1 -> Sum1/1
  Memory/1 -> Sum/2
  Memory1/1 -> Sum2/2
  Gain/1 -> Sum1/2
  S0/1(y) -> S1/1(u)
  Compare To Constant/1 -> Data Type Conversion/1
  Compare To Constant1/1 -> Data Type Conversion1/1
  Sum2/1 -> Memory1/1, Gain1/1
  Sum/1 -> Compare To Constant1/1, Compare To Constant/1
  Sum1/1 -> Sum2/1
  ang/1 -> Sum3/2, Memory/1, Sum/1
  S1/1(y) -> Gain2/1

== system templateVFreplay/VF Replay/GENERATION/GENTPJ_TRANSFORMER/freqMeas ==
  ang : Inport
  Compare To Constant : simulink/Logic and Bit Operations/Compare To Constant  relop=>=  const=1.9*pi  OutDataTypeStr=boolean
  Compare To Constant1 : simulink/Logic and Bit Operations/Compare To Constant  relop=<=  const=-1.9*pi  OutDataTypeStr=boolean
  Constant : Constant  Value=dataSim(l).Fact(1)/Fnom
  Data Type Conversion : DataTypeConversion
  Data Type Conversion1 : DataTypeConversion
  Gain : Gain  Gain=-1
  Gain1 : Gain  Gain=-2*pi
  Gain2 : Gain  Gain=100/(2*pi*Fnom)
  Memory : Memory  InheritSampleTime=on
  Memory1 : Memory  InheritSampleTime=on
  S0 : Subsystem
      mask Display: disp('s T_{w1} / (1 + s T_{w1})','texmode','on');
  S1 : Subsystem
      mask Display: disp('1/ (1 + s T)','texmode','on');
  Sum : Sum  Inputs=+-
  Sum{1..4} (4 alike) : Sum
  freq : Outport  VectorParamsAs1DForOutWhenUnconnected=off
  wires:
  S1/1(y) -> Gain2/1
  ang/1 -> Sum/1, Memory/1, Sum3/2
  Sum1/1 -> Sum2/1
  Sum/1 -> Compare To Constant/1, Compare To Constant1/1
  Sum2/1 -> Gain1/1, Memory1/1
  Compare To Constant1/1 -> Data Type Conversion1/1
  Compare To Constant/1 -> Data Type Conversion/1
  S0/1(y) -> S1/1(u)
  Gain/1 -> Sum1/2
  Memory1/1 -> Sum2/2
  Memory/1 -> Sum/2
  Data Type Conversion/1 -> Sum1/1
  Data Type Conversion1/1 -> Gain/1
  Gain1/1 -> Sum3/1
  Sum3/1 -> S0/1(u)
  Constant/1 -> Sum4/2
  Gain2/1 -> Sum4/1
  Sum4/1 -> freq/1

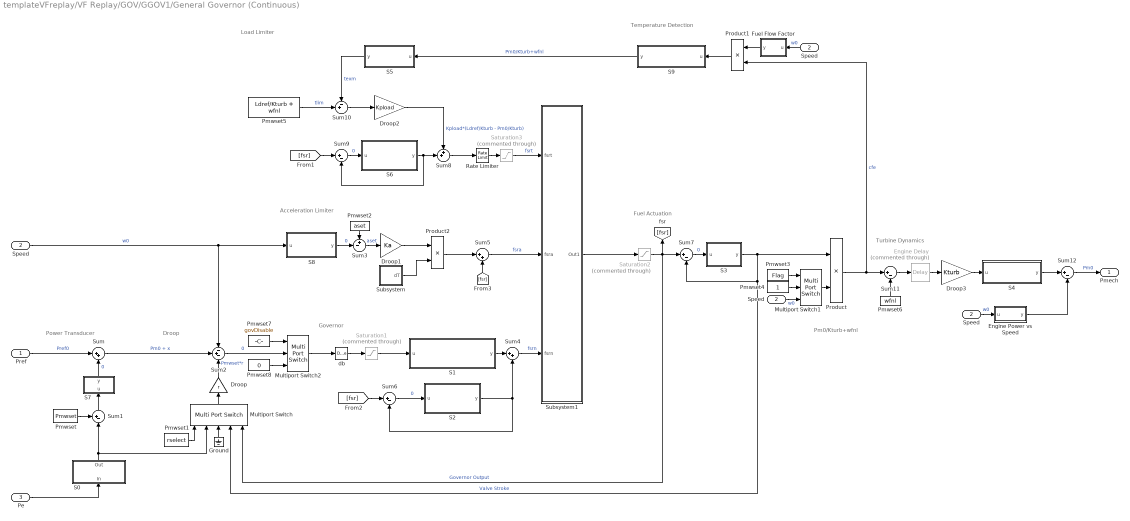
== system templateVFreplay/VF Replay/GOV/GGOV1/General Governor (Continuous)  ==
  note: Acceleration Limiter
  note: Governor
  note: Droop
  note: Power Transducer
  note: Fuel Actuation
  note: Turbine Dynamics
  note: Temperature Detection
  note: Load Limiter
  note: Pm0/Kturb+wfnl
  Pref : Inport
  Speed : Inport  Port=2
  Pe : Inport  Port=3
  " Speed " : InportShadow  Port=2
  Droop : Gain  Gain=r
  Droop1 : Gain  Gain=Ka
  Droop2 : Gain  Gain=Kpload
  Droop3 : Gain  Gain=Kturb
  Engine Delay : TransportDelay  Commented=through  DelayTime=Teng
  Engine Power vs Speed : Subsystem
      mask Display: disp('D_m \times \omega','texmode','on');
  Fuel Flow Factor : Subsystem
      mask Display: disp('\omega^{Dm}','texmode','on');
  Ground : Ground
  Multiport Switch : MultiPortSwitch  Inputs=4
  Multiport Switch1 : MultiPortSwitch  Inputs=2
  Multiport Switch2 : MultiPortSwitch  DataPortOrder=Zero-based contiguous  Inputs=2  zeroidx=on
  Pmwset : Constant  Value=Pmwset
  Pmwset1 : Constant  Value=rselect
  Pmwset2 : Constant  Value=aset
  Pmwset3 : Constant  Value=Flag
  Pmwset4 : Constant
  Pmwset5 : Constant  Value=Ldref/Kturb + wfnl
  Pmwset6 : Constant  Value=wfnl
  Pmwset7 : Constant  Value=govDisable
  Pmwset8 : Constant  Value=0
  Product : Product
  Product1 : Product
  Product2 : Product
  Rate Limiter : RateLimiter  RisingSlewLimit=rup  FallingSlewLimit=rdown  SampleTimeMode=inherited
      settings: AttributesFormatString=|
      | %<RisingSlewLimit>
      | %<FallingSlewLimit>
  S0 : Subsystem
      mask Display: disp('1 / (1 + s T_{pelec})','texmode','on');
  S1 : Subsystem
      mask Display: disp('K_{pgov} + s K_{dgov} / (1 + s T_{dgov})','texmode','on');
  S2 : Subsystem
      mask Display: disp('K_{igov} / (s K_{pgov})','texmode','on');
  S3 : Subsystem
      mask Display: disp('1 / (s T_{act})','texmode','on');
  S4 : Subsystem
      mask Display: disp('(1 + s T_{c}) / (1 + s T_{b})','texmode','on');
  S5 : Subsystem
      mask Display: disp('1 / (1 + s T_{fload})','texmode','on');
  S6 : Subsystem
      mask Display: disp('K_{iload} / (s K_{pload})','texmode','on');
  S7 : Subsystem
      mask Display: disp('K_{imw}/s','texmode','on');
  S8 : Subsystem
      mask Display: disp('s / (1 + s T_a)','texmode','on');
  S9 : Subsystem
      mask Display: disp('(1 + s T_{sa}) / (1 + s T_{sb})','texmode','on');
  Saturation1 : Saturate  Commented=through  UpperLimit=maxerr  LowerLimit=minerr
      settings: AttributesFormatString=|
      | %<UpperLimit>
      | %<LowerLimit>
  Saturation2 : Saturate  Commented=through  UpperLimit=vmax  LowerLimit=vmin
      settings: AttributesFormatString=|
      | %<UpperLimit>
      | %<LowerLimit>
  Saturation3 : Saturate  Commented=through  UpperLimit=1  LowerLimit=-Inf
      settings: AttributesFormatString=|
      | %<UpperLimit>
      | %<LowerLimit>
  "Speed " : InportShadow  Port=2
  "Speed  " : InportShadow  Port=2
  Subsystem : Subsystem
      mask Display: disp('\Delta T','texmode','on');
  Subsystem1 : Subsystem
  Sum : Sum  Inputs=|++
  Sum1 : Sum  Inputs=+-|
  Sum10 : Sum  Inputs=-+|
  Sum{6..7,9,11..12} (5 alike) : Sum  Inputs=|+-
  Sum2 : Sum  Inputs=-+-
  Sum3 : Sum  Inputs=+-|
  Sum4 : Sum  Inputs=|++
  Sum5 : Sum  Inputs=|++
  Sum8 : Sum  Inputs=++|
  db : DeadZone  LowerValue=db  UpperValue=-db  SaturateOnIntegerOverflow=on
  Pmech : Outport  VectorParamsAs1DForOutWhenUnconnected=off
  wires:
  " Speed "/1 -> Engine Power vs Speed/1(u)  "w0"
  Engine Power vs Speed/1(y) -> Sum12/2
  S4/1(y) -> Sum12/1
  Droop3/1 -> S4/1(u)
  Engine Delay/1 -> Droop3/1
  Sum11/1 -> Engine Delay/1
  Pmwset6/1 -> Sum11/2
  Fuel Flow Factor/1(y) -> Product1/1
  "Speed  "/1 -> Fuel Flow Factor/1(u)  "w0"
  Product1/1 -> S9/1(u)
  S9/1(y) -> S5/1(u)  "Pm0/Kturb+wfnl"
  S5/1(y) -> Sum10/1  "texm"
  Pmwset5/1 -> Sum10/2  "tlim"
  Sum10/1 -> Droop2/1
  Droop2/1 -> Sum8/1  "Kpload*(Ldref/Kturb - Pm0/Kturb)"
  S6/1(y) -> Sum9/2, Sum8/2
  Sum9/1 -> S6/1(u)  "0"
  [fsr] -> Sum9/1
  Sum8/1 -> Rate Limiter/1
  Rate Limiter/1 -> Saturation3/1
  Product/1 -> Product1/2, Sum11/1  "cfe"
  "Speed "/1 -> Multiport Switch1/3  "w0"
  Pmwset4/1 -> Multiport Switch1/2
  Pmwset3/1 -> Multiport Switch1/1
  S3/1(y) -> Product/1, Multiport Switch/4, Sum7/2  "Valve Stroke"
  Sum7/1 -> S3/1(u)  "0"
  [fsr] -> Sum5/2
  Sum6/1 -> S2/1(u)  "0"
  S2/1(y) -> Sum6/2, Sum4/2
  [fsr] -> Sum6/1
  Saturation2/1 -> [fsr], Sum7/1, Multiport Switch/5  "Governor Output"
  Sum3/1 -> Droop1/1  "aset"
  S1/1(y) -> Sum4/1
  Saturation1/1 -> S1/1(u)
  db/1 -> Saturation1/1
  Pmwset2/1 -> Sum3/1
  S8/1(y) -> Sum3/2  "0"
  Ground/1 -> Multiport Switch/3
  Pmwset1/1 -> Multiport Switch/1
  Multiport Switch/1 -> Droop/1
  Pe/1 -> S0/1(In)
  S0/1(Out) -> Sum1/2, Multiport Switch/2
  Droop/1 -> Sum2/3  "Pmwset*r"
  Speed/1 -> Sum2/1, S8/1(u)  "w0"
  Sum/1 -> Sum2/2  "Pm0 + x"
  Pmwset/1 -> Sum1/1
  Sum1/1 -> S7/1(u)
  S7/1(y) -> Sum/2  "0"
  Pref/1 -> Sum/1  "Pref0"
  Sum12/1 -> Pmech/1  "Pm0"
  Droop1/1 -> Product2/1
  Product2/1 -> Sum5/1
  Subsystem/1(dT) -> Product2/2
  Subsystem1/1(Out1) -> Saturation2/1
  Multiport Switch1/1 -> Product/2
  Saturation3/1 -> Subsystem1/1(fsrt)  "fsrt"
  Sum5/1 -> Subsystem1/2(fsra)  "fsra"
  Sum4/1 -> Subsystem1/3(fsrn)  "fsrn"
  Multiport Switch2/1 -> db/1
  Pmwset7/1 -> Multiport Switch2/1
  Sum2/1 -> Multiport Switch2/2  "0"
  Pmwset8/1 -> Multiport Switch2/3

== system templateVFreplay/VF Replay/GOV/IEEEG3/Hydro Turbine//Governor (Continuous) ==
  Pref : Inport
  Speed : Inport  Port=2
  Gain1 : Gain  Gain=Rperm
  Gain7 : Gain  Gain=1/Tg
  Integrator : Integrator  LimitOutput=on  UpperSaturationLimit=Pmax  LowerSaturationLimit=Pmin
      settings: AttributesFormatString=|
      | %<UpperSaturationLimit>
      | %<LowerSaturationLimit>
  Pgv : Lookup_n-D  NumberOfTableDimensions=1  BreakpointsForDimension1=[0 Gv 1]  Table=[0 Pgv 1]  InternalRulePriority=Speed  RndMeth=Simplest  InputSameDT=on
  S0 : Subsystem
      mask Display: disp('1/(1+sTp)')
  S2 : Subsystem
      mask Display: disp('R_{temp} s T_r / (1 + s T_r)','texmode','on');
  S3 : Subsystem
      mask Display: disp('R_{turb} (1 + s A_{turb} T_w) / (1 + s B_{turb} T_w)','texmode','on');
  Saturation1 : Saturate  UpperLimit=Uo  LowerLimit=Uc
      settings: AttributesFormatString=|
      | %<UpperLimit>
      | %<LowerLimit>
  Sum : Sum  Inputs=+--
  Sum1 : Sum  Inputs=|++
  db1 : DeadZone  LowerValue=db1  UpperValue=-db1  SaturateOnIntegerOverflow=on
  db2 : Backlash  BacklashWidth=2*db2  ZeroCross=off
  Pmech : Outport  InitialOutput=0  VectorParamsAs1DForOutWhenUnconnected=off
  wires:
  Gain7/1 -> Saturation1/1
  S0/1(y) -> Gain7/1
  Saturation1/1 -> Integrator/1
  Speed/1 -> db1/1
  Pref/1 -> Sum/1  "Pm0"
  db1/1 -> Sum/2
  Gain1/1 -> Sum1/2
  S3/1(y) -> Pmech/1
  Sum/1 -> S0/1(u)
  S2/1(y) -> Sum1/1
  Integrator/1 -> db2/1
  Sum1/1 -> Sum/3
  Pgv/1 -> S3/1(u)
  db2/1 -> Pgv/1, S2/1(u), Gain1/1  "Gv0"

== system templateVFreplay/VF Replay/PSS/PSS1A/Power System Stabilize 1A (Continuous) ==
  Input : Inport
  (ta.s+1)/(tb.s+1) : modelLibrary/(ta.s+1)//(tb.s+1)  ta=T1  tb=T2
  (ta.s+1)/(tb.s+1)1 : Subsystem  mask{ta=T3, tb=T4}
      mask prompts: ta "numerator tau (ta)"; tb "denominator tau  (tb)"
  S3_1 : Subsystem
      mask Display: disp('1/(1+sA1 + s^2 A2)')
  Saturation2 : Saturate  UpperLimit=Vrmax  LowerLimit=Vrmin
      settings: AttributesFormatString=|
      | %<UpperLimit>
      | %<LowerLimit>
  k.tau.s/(tau.s+1) : modelLibrary/k.tau.s//(tau.s+1)  k=Ks  tau=T5
  k/(tau.s+1) : modelLibrary/k//(tau.s+1)  k=1  tau=T6  vmax=Inf  vmin=-Inf
  Vstab : Outport  VectorParamsAs1DForOutWhenUnconnected=off
  wires:
  k.tau.s/(tau.s+1)/1 -> S3_1/1(u)
  S3_1/1(y) -> (ta.s+1)/(tb.s+1)/1
  k/(tau.s+1)/1 -> k.tau.s/(tau.s+1)/1
  Input/1 -> k/(tau.s+1)/1
  (ta.s+1)/(tb.s+1)/1 -> (ta.s+1)/(tb.s+1)1/1(u)
  (ta.s+1)/(tb.s+1)1/1(y) -> Saturation2/1
  Saturation2/1 -> Vstab/1

== system templateVFreplay/VF Replay/PSS/PSS2A/Power System Stabilizer 2A (Continuous)  ==
  Input_1 : Inport
  Input_2 : Inport  Port=2
  (T1.s+1)/(T2.s+1) : modelLibrary/(ta.s+1)//(tb.s+1)  ta=T1  tb=T2
  (T3.s+1)/(T4.s+1) : modelLibrary/(ta.s+1)//(tb.s+1)  ta=T3  tb=T4
  (ta.s+a)/(tb.s+1) : modelLibrary/(ta.s+a)//(tb.s+1)  ta=Ta  tb=Tb  a=a
  Ks1 : Gain  Gain=Ks4
  Ks2 : Gain  Gain=Ks1
  Ks3 : Gain  Gain=Ks3
  Saturation2 : Saturate  Commented=through  UpperLimit=Vstmax  LowerLimit=Vstmin
      settings: AttributesFormatString=|
      | %<UpperLimit>
      | %<LowerLimit>
  Sum : Sum  Inputs=|++
  Sum1 : Sum  Inputs=|+-
  T9 ~= 0 : Subsystem  VariantControl=T9NotZero  mask{M=M, N=N, T8=T8, T9=T9}
      mask prompts: M "M, Denominator Order"; N "N, Number of Series Filters"; T8 "T8, Lead Ramp Tracking Constant [s]"; T9 "T9, Lag Ramp Tracking Constant [s]"
      mask Display: disp('[(1 + s T_8) / (1 + s T_9)^m]^n','texmode','on');
  Tw1.s/(Tw1.s+1) : modelLibrary/k.s//(tau.s+1)  k=Tw1  tau=Tw1
  Tw2.s/(Tw2.s+1) : modelLibrary/k.s//(tau.s+1)  k=Tw2  tau=Tw2
  Tw3.s/(Tw3.s+1) : modelLibrary/k.s//(tau.s+1)  k=Tw3  tau=Tw3
  Tw4.s/(Tw4.s+1) : modelLibrary/k.s//(tau.s+1)  k=Tw4  tau=Tw4
  k/(tau.s+1) : modelLibrary/k//(tau.s+1)  k=Ks2  tau=T7  vmax=Inf  vmin=-Inf
  Vstab : Outport  VectorParamsAs1DForOutWhenUnconnected=off
  wires:
  Tw4.s/(Tw4.s+1)/1 -> k/(tau.s+1)/1
  Tw3.s/(Tw3.s+1)/1 -> Tw4.s/(Tw4.s+1)/1
  Input_2/1 -> Tw3.s/(Tw3.s+1)/1
  Input_1/1 -> Tw1.s/(Tw1.s+1)/1
  Tw1.s/(Tw1.s+1)/1 -> Tw2.s/(Tw2.s+1)/1
  Tw2.s/(Tw2.s+1)/1 -> Sum/1
  k/(tau.s+1)/1 -> Ks1/1, Ks3/1
  Ks3/1 -> Sum/2
  Ks1/1 -> Sum1/2
  Sum1/1 -> Ks2/1
  Sum/1 -> T9 ~= 0/1(u)
  T9 ~= 0/1(y) -> Sum1/1
  Saturation2/1 -> Vstab/1
  Ks2/1 -> (T1.s+1)/(T2.s+1)/1
  (T1.s+1)/(T2.s+1)/1 -> (T3.s+1)/(T4.s+1)/1
  (T3.s+1)/(T4.s+1)/1 -> (ta.s+a)/(tb.s+1)/1
  (ta.s+a)/(tb.s+1)/1 -> Saturation2/1

== system templateVFreplay/VF Replay/PSS/PSS2B/Power System Stabilizer 2B (Continuous)  ==
  Input_1 : Inport
  Input_2 : Inport  Port=2
  (T1.s+1)/(T2.s+1) : modelLibrary/(ta.s+1)//(tb.s+1)  ta=T1  tb=T2
  (T3.s+1)/(T4.s+1) : modelLibrary/(ta.s+1)//(tb.s+1)  ta=T3  tb=T4
  (ta.s+a)/(tb.s+1) : modelLibrary/(ta.s+a)//(tb.s+1)  ta=Ta  tb=Tb  a=a
  Ks1 : Gain  Gain=Ks4
  Ks2 : Gain  Gain=Ks1
  Ks3 : Gain  Gain=Ks3
  Saturation2 : Saturate  Commented=through  UpperLimit=Vstmax  LowerLimit=Vstmin
      settings: AttributesFormatString=|
      | %<UpperLimit>
      | %<LowerLimit>
  Sum : Sum  Inputs=|++
  Sum1 : Sum  Inputs=|+-
  T9 ~= 0 : Subsystem  VariantControl=T9NotZero  mask{M=M, N=N, T8=T8, T9=T9}
      mask prompts: M "M, Denominator Order"; N "N, Number of Series Filters"; T8 "T8, Lead Ramp Tracking Constant [s]"; T9 "T9, Lag Ramp Tracking Constant [s]"
      mask Display: disp('[(1 + s T_8) / (1 + s T_9)^m]^n','texmode','on');
  Tw1.s/(Tw1.s+1) : modelLibrary/k.s//(tau.s+1)  k=Tw1  tau=Tw1
  Tw2.s/(Tw2.s+1) : modelLibrary/k.s//(tau.s+1)  k=Tw2  tau=Tw2
  Tw3.s/(Tw3.s+1) : modelLibrary/k.s//(tau.s+1)  k=Tw3  tau=Tw3
  Tw4.s/(Tw4.s+1) : modelLibrary/k.s//(tau.s+1)  k=Tw4  tau=Tw4
  k/(tau.s+1) : modelLibrary/k//(tau.s+1)  k=Ks2  tau=T7  vmax=Inf  vmin=-Inf
  Vstab : Outport  VectorParamsAs1DForOutWhenUnconnected=off
  wires:
  Tw4.s/(Tw4.s+1)/1 -> k/(tau.s+1)/1
  Tw3.s/(Tw3.s+1)/1 -> Tw4.s/(Tw4.s+1)/1
  Input_2/1 -> Tw3.s/(Tw3.s+1)/1
  Input_1/1 -> Tw1.s/(Tw1.s+1)/1
  Tw1.s/(Tw1.s+1)/1 -> Tw2.s/(Tw2.s+1)/1
  Tw2.s/(Tw2.s+1)/1 -> Sum/1
  k/(tau.s+1)/1 -> Ks1/1, Ks3/1
  Ks3/1 -> Sum/2
  Ks1/1 -> Sum1/2
  Sum1/1 -> Ks2/1
  Sum/1 -> T9 ~= 0/1(u)
  T9 ~= 0/1(y) -> Sum1/1
  Saturation2/1 -> Vstab/1
  Ks2/1 -> (T1.s+1)/(T2.s+1)/1
  (T1.s+1)/(T2.s+1)/1 -> (T3.s+1)/(T4.s+1)/1
  (T3.s+1)/(T4.s+1)/1 -> (ta.s+a)/(tb.s+1)/1
  (ta.s+a)/(tb.s+1)/1 -> Saturation2/1

== system templateVFreplay/VF Replay/AVR/REXS/Rotating Excitation System (Continuous) /S1 ==
  u : Inport
  Gain1 : Gain  Gain=Kvi
  Gain7 : Gain  Gain=Kvp
  Integrator : Integrator
  Sum : Sum  Inputs=|++
  y : Outport  InitialOutput=0  VectorParamsAs1DForOutWhenUnconnected=off
  wires:
  Sum/1 -> y/1
  Integrator/1 -> Sum/2
  Gain7/1 -> Sum/1
  Gain1/1 -> Integrator/1
  u/1 -> Gain7/1, Gain1/1

== system templateVFreplay/VF Replay/AVR/REXS/Rotating Excitation System (Continuous) /S2 + S8 ==
  u : Inport
  S2 : Subsystem  VariantControlMode=Label  Variant=on  LabelModeActiveChoice=Tb1NotZero
      mask Display: disp('(1 + s T_{c1}) / (1 + s T_{b1})','texmode','on');
  S8 : Subsystem  VariantControlMode=Label  Variant=on  LabelModeActiveChoice=Tb2NotZero
      mask Display: disp('(1 + s T_{c2}) / (1 + s T_{b2})','texmode','on');
  y : Outport  InitialOutput=0  VectorParamsAs1DForOutWhenUnconnected=off
  wires:
  u/1 -> S2/1(In)
  S2/1(Out) -> S8/1(In)
  S8/1(Out) -> y/1

== system templateVFreplay/VF Replay/AVR/REXS/Rotating Excitation System (Continuous) /S5 ==
  u : Inport
  Gain : Gain  Gain=1/Tf
  Gain1 : Gain  Gain=Kf
  Integrator : Integrator
  Sum : Sum  Inputs=|+-
  y : Outport  InitialOutput=0  VectorParamsAs1DForOutWhenUnconnected=off
  wires:
  Gain1/1 -> y/1
  u/1 -> Sum/1
  Sum/1 -> Gain/1
  Integrator/1 -> Sum/2
  Gain/1 -> Integrator/1, Gain1/1

== system templateVFreplay/VF Replay/AVR/REXS/Rotating Excitation System (Continuous) /S6 ==
  u : Inport
  Gain1 : Gain  Gain=Kii
  Gain7 : Gain  Gain=Kip
  Integrator : Integrator
  Sum : Sum  Inputs=|++
  y : Outport  InitialOutput=0  VectorParamsAs1DForOutWhenUnconnected=off
  wires:
  u/1 -> Gain1/1, Gain7/1
  Gain1/1 -> Integrator/1
  Gain7/1 -> Sum/1
  Integrator/1 -> Sum/2
  Sum/1 -> y/1

== system templateVFreplay/VF Replay/AVR/REXS/Rotating Excitation System (Continuous) /S7 ==
  u : Inport
  Gain1 : Gain  Gain=1/Te
  Integrator : Integrator  InitialCondition=1  LimitOutput=on  LowerSaturationLimit=0
  y : Outport  InitialOutput=0  VectorParamsAs1DForOutWhenUnconnected=off
  wires:
  u/1 -> Gain1/1
  Gain1/1 -> Integrator/1
  Integrator/1 -> y/1

== system templateVFreplay/VF Replay/AVR/REXS/Rotating Excitation System (Continuous) /Scaling ==
  note: In<=0.433        Case 3
      | 0.433<In<0.75 Case 2
      | 0.75<=In<=1.0 Case 1
      | In>1.0               default
  note: Rectifier regulation equations
  note: In=Kc*Ifd/Ve
  Ve : Inport
  Ifd : Inport  Port=2
  0.433<In<0.75 : spsST2AModel/Continuous/Rectifier/0.433<In<0.75  SystemSampleTime=-1  Latency=0  AutoFrameSizeCalculation=off
      settings: SourceProductName=Simscape Electrical  SourceProductBaseCode=PS
  0.75<=In<=1.0 : spsST2AModel/Continuous/Rectifier/0.75<=In<=1.0  SystemSampleTime=-1  Latency=0  AutoFrameSizeCalculation=off
      settings: SourceProductName=Simscape Electrical  SourceProductBaseCode=PS
  Fcn : Fcn  Expr=u+(u==0)*eps
  Gain : Gain  Gain=Kc  SaturateOnIntegerOverflow=on  OutDataTypeStr=Inherit: Same as input  ParamDataTypeStr=Inherit: Same as input
  In<=0.433 : spsST2AModel/Continuous/Rectifier/In<=0.433  SystemSampleTime=-1  Latency=0  AutoFrameSizeCalculation=off
      settings: SourceProductName=Simscape Electrical  SourceProductBaseCode=PS
  In>1.0 : spsST2AModel/Continuous/Rectifier/In>1.0  SystemSampleTime=-1  Latency=0  AutoFrameSizeCalculation=off
      settings: SourceProductName=Simscape Electrical  SourceProductBaseCode=PS
  Merge : Merge  Inputs=4
  Product : Product  Inputs=*/  SaturateOnIntegerOverflow=on  RndMeth=Zero  InputSameDT=on  OutDataTypeStr=Inherit: Same as first input
  Relational Operator : RelationalOperator  Operator=<=  RndMeth=Nearest  InputSameDT=on
  Relational Operator1 : RelationalOperator  Operator=<  RndMeth=Nearest  InputSameDT=on
  Relational Operator2 : RelationalOperator  Operator=<=  RndMeth=Nearest  InputSameDT=on
  Sum : Sum  Inputs=+++  AccumDataTypeStr=double  OutDataTypeStr=double  SaturateOnIntegerOverflow=on  InputSameDT=on
  Switch Case : SwitchCase  CaseConditions={1 2 3}
  input : Constant  Value=0.433
  input1 : Constant  Value=0.75
  input2 : Constant  Value=1.0
  Fex : Outport  VectorParamsAs1DForOutWhenUnconnected=off
  wires:
  Ve/1 -> Fcn/1
  Fcn/1 -> Product/2
  Ifd/1 -> Product/1
  Product/1 -> Gain/1
  Gain/1 -> Relational Operator2/1, 0.433<In<0.75/1, 0.75<=In<=1.0/1, In<=0.433/1, Relational Operator1/1, Relational Operator/1  "In"
  Merge/1 -> Fex/1
  0.75<=In<=1.0/1 -> Merge/1
  0.433<In<0.75/1 -> Merge/2
  In>1.0/1 -> Merge/4
  In<=0.433/1 -> Merge/3
  input1/1 -> Relational Operator1/2
  input2/1 -> Relational Operator2/2
  Relational Operator1/1 -> Sum/2
  Relational Operator/1 -> Sum/1
  Relational Operator2/1 -> Sum/3
  Sum/1 -> Switch Case/1
  Switch Case/1 -> 0.75<=In<=1.0/Action
  Switch Case/2 -> 0.433<In<0.75/Action
  Switch Case/3 -> In<=0.433/Action
  Switch Case/4 -> In>1.0/Action
  input/1 -> Relational Operator/2

== system templateVFreplay/VF Replay/AVR/REXS/Rotating Excitation System (Continuous) /Scaling1 ==
  Ve : Inport
  1-D Lookup Table : Lookup_n-D  NumberOfTableDimensions=1  BreakpointsForDimension1=[0 E(1) E(2)]  Table=[0 Se(1) Se(2)]  InternalRulePriority=Speed  RndMeth=Simplest  InputSameDT=on
  Product1 : Product  RndMeth=Zero
  Sum : Sum  Inputs=++|
  Xc4 : Gain  Gain=Ke
  Vx : Outport  VectorParamsAs1DForOutWhenUnconnected=off
  wires:
  Xc4/1 -> Sum/1
  Product1/1 -> Sum/2
  1-D Lookup Table/1 -> Product1/2  "Se[Ve]"
  Ve/1 -> Product1/1, 1-D Lookup Table/1, Xc4/1
  Sum/1 -> Vx/1

== system templateVFreplay/VF Replay/AVR/REXS/Rotating Excitation System (Continuous) /Ta ~= 0 ==
  In : Inport
  1/Ta : Gain  Gain=1/Ta
  Integrator : Integrator  InitialCondition=0.5  LimitOutput=on  UpperSaturationLimit=Vrmax  LowerSaturationLimit=Vrmin
  Sum : Sum  Inputs=|+-
  Out : Outport  InitialOutput=0  VectorParamsAs1DForOutWhenUnconnected=off
  wires:
  Sum/1 -> 1/Ta/1
  1/Ta/1 -> Integrator/1
  In/1 -> Sum/1
  Integrator/1 -> Sum/2, Out/1

== system templateVFreplay/VF Replay/AVR/REXS/Rotating Excitation System (Continuous) /Tf2 ~= 0 ==
  In : Inport
  Gain : Gain  Gain=1/Tf2
  Gain1 : Gain  Gain=Tf1
  Integrator : Integrator
  Sum : Sum  Inputs=|+-
  Sum1 : Sum  Inputs=++|
  Out : Outport  InitialOutput=0  VectorParamsAs1DForOutWhenUnconnected=off
  wires:
  Gain1/1 -> Sum1/1
  Integrator/1 -> Sum/2, Sum1/2
  Sum/1 -> Gain/1
  Gain/1 -> Integrator/1, Gain1/1
  Sum1/1 -> Out/1
  In/1 -> Sum/1

== system templateVFreplay/VF Replay/AVR/REXS/Rotating Excitation System (Continuous) /Tr ~= 0 ==
  In : Inport
  1/Tr : Gain  Gain=1/Tr
  Integrator : Integrator
  Sum : Sum  Inputs=|+-
  Out : Outport  InitialOutput=0  VectorParamsAs1DForOutWhenUnconnected=off
  wires:
  Sum/1 -> 1/Tr/1
  1/Tr/1 -> Integrator/1
  In/1 -> Sum/1
  Integrator/1 -> Sum/2, Out/1

== system templateVFreplay/VF Replay/AVR/ST1A/ST1A Excitation System/Model ==
  note: Efd0
  note: Efd0
  note: VA0/Ka
  note: VA0/Ka
  note: Vt.VRmin
  note: VA0/Ka
  note: Efd0
  note: 0
  note: Vt0
  note: Vt.VRmax-Kc.Ifd
  note: Main Regulator
      | Ka/(Ta.s+1)
  note: VImax
  note: Initial values are shown in blue
  note: Vt0
  note: __
      |              /
      |           /
      |         /
      |       /
      | __/
  note: Limits VImin, VImax
  note: VAmax
  note: VAmin
  note: VA0/Ka
  note: KLR*(Ifd-ILR)
  note: VA0=Efd0+KLR*(Ifd-ILR)
  note: VA0
  note: Vt0
  Vref : Inport
  Vt : Inport  Port=2
  Ifd : Inport  Port=3
  Vstab : Inport  Port=4
  (ta.s+1)/(tb.s+1) : modelLibrary/(ta.s+1)//(tb.s+1)  ta=Tc  tb=Tb
  (ta.s+1)/(tb.s+1)1 : Subsystem  mask{ta=Tc1, tb=Tb1}
      mask prompts: ta "numerator tau (ta)"; tb "denominator tau  (tb)"
  ILR : Constant  Value=p.ilr
  KLR : Gain  Gain=p.klr  SaturateOnIntegerOverflow=on  OutDataTypeStr=Inherit: Same as input  ParamDataTypeStr=Inherit: Same as input
  Subsystem : Subsystem
      mask Display: plot([0.15 0.85],[.5 .5],[.5 .5],[0.05 0.95],0.15+0.7*[0 .25 .75 1],0.05+0.9*[.25 .25 .75 .75]);
  Sum : Sum  Inputs=++-+-  SaturateOnIntegerOverflow=on  InputSameDT=on  OutDataTypeStr=Inherit: Same as first input
  Sum1 : Sum  Inputs=|+-  SaturateOnIntegerOverflow=on  InputSameDT=on  OutDataTypeStr=Inherit: Same as first input
  Sum2 : Sum  Inputs=|+-  SaturateOnIntegerOverflow=on  InputSameDT=on  OutDataTypeStr=Inherit: Same as first input
  VImin : Saturate  UpperLimit=p.vimax  LowerLimit=p.vimin
  VImin2 : Saturate  UpperLimit=inf  LowerLimit=0
  const : Subsystem
  k.s/(tau.s+1) : Subsystem  mask{k=Kf, tau=Tf}
  k/(tau.s+1) : modelLibrary/k//(tau.s+1)  k=1  tau=p.tr  vmax=Inf  vmin=-Inf
  k/(tau.s+1)1 : Subsystem  mask{k=p.ka, tau=p.ta, vmax=p.vamax, vmin=p.vamin}
  Efd : Outport  VectorParamsAs1DForOutWhenUnconnected=off
  wires:
  Ifd/1 -> Sum1/1, Subsystem/3(Ifd)
  Subsystem/1(Efd1) -> Efd/1  "Efd"
  Vt/1 -> k/(tau.s+1)/1  "Vt"
  k/(tau.s+1)1/1(y) -> Sum2/1  "VA"
  Sum/1 -> VImin/1
  Sum1/1 -> KLR/1
  ILR/1 -> Sum1/2
  Sum2/1 -> k.s/(tau.s+1)/1(u), Subsystem/1(Efd)  "Efd"
  (ta.s+1)/(tb.s+1)1/1(y) -> k/(tau.s+1)1/1(u)
  KLR/1 -> VImin2/1
  Vref/1 -> Sum/1
  k/(tau.s+1)/1 -> Sum/3, Subsystem/2(Vt)  "Vt"
  VImin2/1 -> Sum2/2
  k.s/(tau.s+1)/1(y) -> Sum/5  "Vf"
  VImin/1 -> (ta.s+1)/(tb.s+1)/1  "VI"
  Vstab/1 -> Sum/4
  const/1(y) -> Sum/2
  (ta.s+1)/(tb.s+1)/1 -> (ta.s+1)/(tb.s+1)1/1(u)

== system templateVFreplay/VF Replay/AVR/ST4B/ST4B Excitation System (Continuous)/Break Algebraic Loop  ==
  In : Inport
  1/Tau : Gain  Gain=1/1e-3
  Integrator : Integrator  InitialCondition=1
  Sum : Sum  Inputs=|+-
  Out : Outport  InitialOutput=0  VectorParamsAs1DForOutWhenUnconnected=off
  wires:
  Integrator/1 -> Out/1, Sum/2
  In/1 -> Sum/1
  1/Tau/1 -> Integrator/1
  Sum/1 -> 1/Tau/1
